simulink model "Stateflow_AC"  (R2024b)
settings: Solver=VariableStepAuto  StartTime=0.0  StopTime=inf  RelTol=1e-3
settings Model: Creator=sudee  LastModifiedBy=sudee

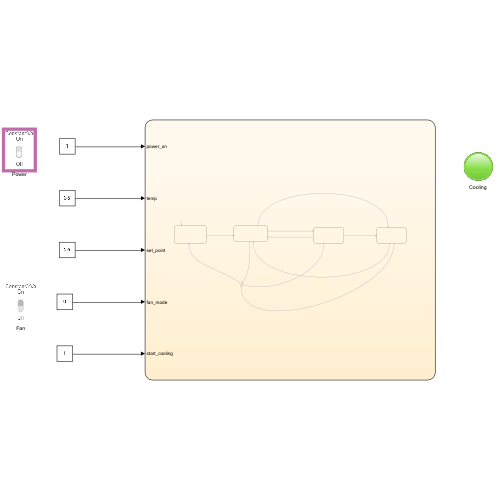
[thumbnail: Simulink's stored preview of the top-level diagram]
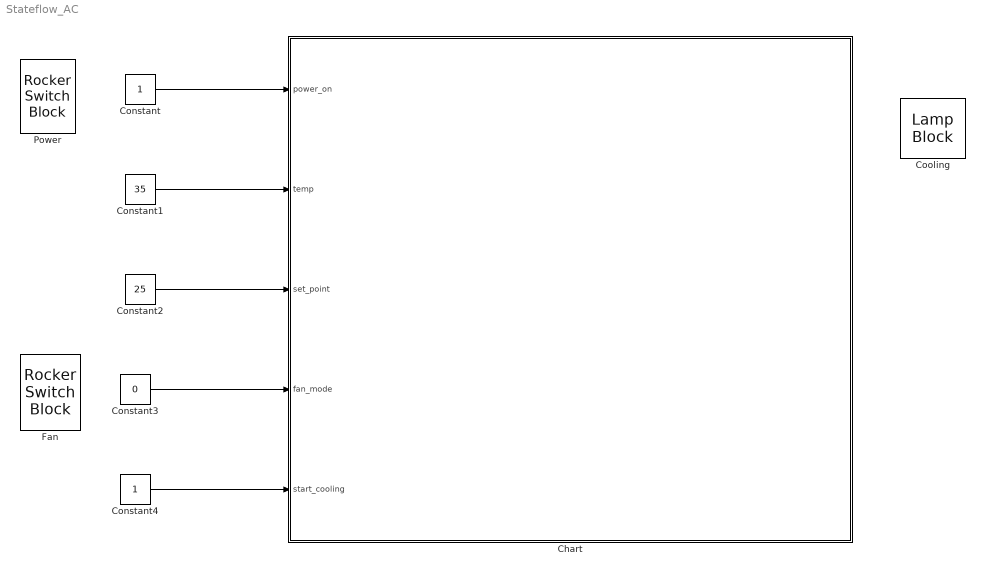
== system Stateflow_AC ==
  Chart : Stateflow chart  TreatAsAtomicUnit=on
  Constant : Constant
  Constant1 : Constant  Value=35
  Constant2 : Constant  Value=25
  Constant3 : Constant  Value=0
  Constant4 : Constant
  Cooling : LampBlock  LabelPosition=Hide
  Fan : RockerSwitchBlock
      settings: Values={{'Off', 'On'}, [0 1]}
  Power : RockerSwitchBlock
      settings: Values={{'Off', 'On'}, [0 1]}
  wires:
  Constant/1 -> Chart/1(power_on)
  Constant1/1 -> Chart/2(temp)
  Constant2/1 -> Chart/3(set_point)
  Constant3/1 -> Chart/4(fan_mode)
  Constant4/1 -> Chart/5(start_cooling)

== stateflow chart Stateflow_AC/Chart ==
  state Off
    entry:
    stop_fan_and_cooling();
  state Standby
    entry:
    stop_fan_and_cooling();
  state Cooling
    entry:
    start_cooling();
    during:
    monitor_temperature();
  state Fan_only
    entry:
    start_fan();
  Standby -> Fan_only [order 2] : [fan_mode == true]
  (default) -> Off
  Standby -> Cooling [order 1] : [temp > set_point]
  Off -> Standby : [power_on == true]
  Cooling -> Fan_only [order 2] : [fan_mode==true]
  Cooling -> Standby [order 1] : [temp<= set_point]
  Standby -> (junction 14) [order 3] : [power_on == false]
  Fan_only -> Standby [order 1] : [fan_mode == false]
  (junction 14) -> Off : [power_on == false]
  Fan_only -> (junction 14) [order 2] : [power_on == false]
  Cooling -> (junction 14) [order 3] : [power_on == false]
  data: power_on input; temp input; set_point input; fan_mode input; monitor_temperature constant double; stop_fan_and_cooling constant double; start_fan constant double; start_cooling input double
